simulink model "Calibration_IcestorageModel"  (R2018b)
settings: Solver=ode45  StartTime=(-31+16)*24*3600*0  StopTime=(31+29+31+30+31+30+31+31)*24*3600 %23*24*3600  EnableMultiTasking=on
libraries: carnot x43
(part 1 of 2)
settings Model: SimulationMode=accelerator  Creator=drhf  LastModifiedBy=drhf
settings DataIOCC: SaveFormat=Array  SignalLoggingSaveFormat=ModelDataLogs  SaveOutput=off  SignalLogging=off  DSMLogging=off  SaveTime=off
settings OptimizationCC: ExpressionDepthLimit=2147483647  LifeSpan=inf
settings DebuggingCC: UnderspecifiedInitializationDetection=Classic  MergeDetectMultiDrivingBlocksExec=none  SolverPrmCheckMsg=warning  FcnCallInpInsideContextMsg=warning  StateNameClashWarn=warning  SFUnexpectedBacktrackingDiag=warning  SFNoUnconditionalDefaultTransitionDiag=warning  SFExecutionAtInitializationDiag=none
settings HardwareCC: ProdBitPerPointer=32  ProdBitPerSizeT=32  ProdBitPerPtrDiffT=32  ProdLargestAtomicFloat=None  ProdIntDivRoundTo=Undefined  ProdEndianess=Unspecified  ProdWordSize=32  ProdHWDeviceType=32-bit Generic
settings ModelReferenceCC: PropagateSignalLabelsOutOfModel=off
settings SFSimCC: SimUseLocalCustomCode=off
settings RTWCC: RTWUseLocalCustomCode=off
settings CodeAppCC: StateflowObjectComments=on
settings GRTTargetCC: TargetLangStandard=C89/C90 (ANSI)  GeneratePreprocessorConditionals=Disable all  CombineOutputUpdateFcns=off  GRTInterface=on
settings ConfigComp: CovMetricSettings=dw  CovHtmlReporting=on  CovSaveCumulativeToWorkspaceVar=on  CovSaveSingleToWorkspaceVar=on  CovExternalEMLEnable=off

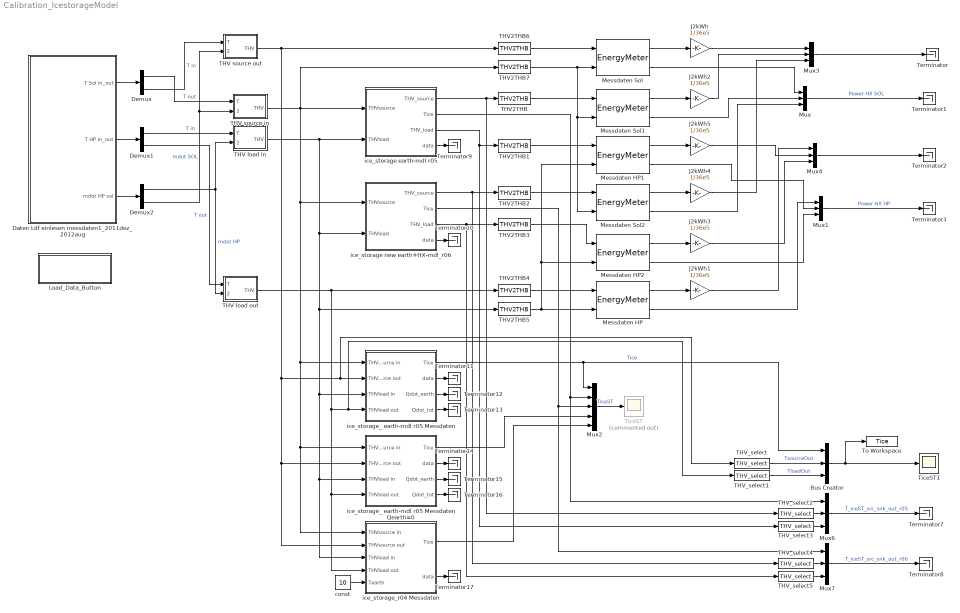
== system Calibration_IcestorageModel ==
  Bus Creator : BusCreator  Inputs=3
  Daten Ldf einlesen messdaten1_2011dez_2012aug : Subsystem
  Demux : Demux  Outputs=2
  Demux1 : Demux  Outputs=2
  Demux2 : Demux  Outputs=2
  J2kWh{,1..5} (6 alike) : Gain  Gain=1/36e5  SaturateOnIntegerOverflow=on  OutDataTypeStr=Inherit: Same as input  ParamDataTypeStr=Inherit: Same as input
  Load_Data_Button : Subsystem
      settings: OpenFcn=|
      | [filename, pathname, filterindex] = ...
      |    uigetfile( {'*.mat','MAT-files (*.mat)'; ...
      |    '*.*',  'All Files (*.*)'},  'Pick a data file');
      | 
      | if (filterindex > 0)
      |    load(filename)
      | end
      mask Display: disp('double click \nto load data')
  Messdaten HP : carnot/Control/EnergyMeter
      settings: SourceProductName=Carnot
  Messdaten HP1 : carnot/Control/EnergyMeter
      settings: SourceProductName=Carnot
  Messdaten HP2 : carnot/Control/EnergyMeter
      settings: SourceProductName=Carnot
  Messdaten Sol : carnot/Control/EnergyMeter
      settings: SourceProductName=Carnot
  Messdaten Sol1 : carnot/Control/EnergyMeter
      settings: SourceProductName=Carnot
  Messdaten Sol2 : carnot/Control/EnergyMeter
      settings: SourceProductName=Carnot
  Mux{,1,3..4,6..7} (6 alike) : Mux  Inputs=3
  Mux2 : Mux  Inputs=5
  THV load in : Subsystem  mask(create THV){p=1e5, fluid=water_glycol_mix, mix=0.5, dia=0.025}
      mask prompts: p "pressure [Pa]"; mix "fluid mixture [0..1]"; dia "diameter [m]"
      mask help: Block to create a THV vector with the variable input T and mdot. The other value can be set as constants in the mask.
      mask init:
      | mix = min(1, max(0, mix));
      | dia = max(dia, 0.001);
      mask Help: eval('man (''create_THV'')')
      mask TypeOptions fluid: water | air | cotton_oil | silicone_oil | water_glycol_mix
  THV load out : Subsystem  mask(create THV){p=1e5, fluid=water_glycol_mix, mix=0.5, dia=0.025}
      mask prompts: p "pressure [Pa]"; mix "fluid mixture [0..1]"; dia "diameter [m]"
      mask help: Block to create a THV vector with the variable input T and mdot. The other value can be set as constants in the mask.
      mask init:
      | mix = min(1, max(0, mix));
      | dia = max(dia, 0.001);
      mask Help: eval('man (''create_THV'')')
      mask TypeOptions fluid: water | air | cotton_oil | silicone_oil | water_glycol_mix
  THV source in : Subsystem  mask(create THV){p=1e5, fluid=water_glycol_mix, mix=0.5, dia=0.025}
      mask prompts: p "pressure [Pa]"; mix "fluid mixture [0..1]"; dia "diameter [m]"
      mask help: Block to create a THV vector with the variable input T and mdot. The other value can be set as constants in the mask.
      mask init:
      | mix = min(1, max(0, mix));
      | dia = max(dia, 0.001);
      mask Help: eval('man (''create_THV'')')
      mask TypeOptions fluid: water | air | cotton_oil | silicone_oil | water_glycol_mix
  THV source out : Subsystem  mask(create THV){p=1e5, fluid=water_glycol_mix, mix=0.5, dia=0.025}
      mask prompts: p "pressure [Pa]"; mix "fluid mixture [0..1]"; dia "diameter [m]"
      mask help: Block to create a THV vector with the variable input T and mdot. The other value can be set as constants in the mask.
      mask init:
      | mix = min(1, max(0, mix));
      | dia = max(dia, 0.001);
      mask Help: eval('man (''create_THV'')')
      mask TypeOptions fluid: water | air | cotton_oil | silicone_oil | water_glycol_mix
  THV2THB{,1..7} (8 alike) : carnot/Toolbox/THV2THB
      settings: SourceProductName=Carnot
  THV_select{,1..5} (6 alike) : carnot/Outputs/THV_select  f=off  t=on  m=off  p=off  id=off  mix=off  d=off  dpcon=off  dplin=off  dpqua=off
      settings: SourceProductName=Carnot
  Terminator{,1..3,7..17} (15 alike) : Terminator
  TiceST : Scope  Commented=on
  TiceST1 : Scope
  To Workspace : ToWorkspace  VariableName=Tice  SaveFormat=Timeseries  SampleTime=600
  const : Constant  Value=10
  ice_storage earth-mdl r05 : Subsystem  mask(simple water storage){vol=10, l_solar=30*3, l_hp=8*40, f_ice=0.075, t_ini=0, z=3.32-0.12, h=2.3, dearth=1, Tmeanoutside=11, deltathetae=9.3, Tmeaninside=5, deltathetai=15, tshift=319 %+8760/2 %to get the right behaviour!, cond_ground=2, cp_ground=800, rho_ground=2500}
      mask prompts: vol "volume [m³]"; l_solar "length of solar heat exchanger [m]"; l_hp "length of HP heat exchanger [m]"; f_ice "Initial fraction of ice (0..1)"; t_ini "Initial Temperatur (only if fraction ice = 0) [°C]"; z "depth of baseplate from upper surface [m]"; h "height of ice storage [m]"; dearth "thickness of surrounding earth layer [m]"; Tmeanoutside "mean outside temperature over one year [°C]"; deltathetae "amplitude of monthly outside temperatures [°C]"; Tmeaninside "mean inside temperature over one year [°C]"; deltathetai "amplitude of monthly mean inside temperature [°C]"; tshift "time shift where external temperature sine-curve shows a minimum [h]"; cond_ground "conductivity of ground [W/(m*K)]"; cp_ground "capacity of ground [J/(kg*K)]"; rho_ground "density of ground [kg/m^3]"
      mask help: multinode water storage
      mask init:
      | f_ice = min(1, max(0, f_ice));
      | h_ini = (1-f_ice)*335e3;
      | if f_ice == 0 
      |     h_ini = h_ini + 4182*t_ini;
      | end
      | %Durchmesser Eisspeicher [m]
      | D_tank = 2.7;
      | %Höhe Eisspeicher [m]
      | h_tank = 2.3;
      | %Grundfläche [m^2]
      | A = pi*(D_tank/2.)^2;
      | %Umfang [m]
      | P = D_tank*pi;
      | %charakteristisches Bodenmass [m]
      | B = A/(0.5*P);
      | %Wärmewiderstand Boden & Wand [m^2*K/W]
      | Rbtot = 0.12/1.330;
      | Rwtot = 0.1/1.330;
      | %Wanddicke [m]
      | w = 0.1;
      | %wirksame Dicke Boden & Wand [m]
      | dt = w + cond_ground*Rbtot;
      | dw = cond_ground*Rwtot;
      | %abstand der mitte der wandfläche zur oberfläche [m]
      | ztilde = z-(0.5*h);
      | %anzahl stunden pro jahr
      | t0 = 8760;
      | %thermische eindringtiefe
      | delta_grd = sqrt((t0*3600*cond_ground)/(pi*rho_ground*cp_ground));
      | 
      | %U-Wert Erdschicht [W/m^2K]
      | U_earth = cond_ground/dearth;
      | %Oberfläche Erdschicht [m^2]
      | A_earth = ((D_tank+2*dearth)/2)^2*pi + (D_tank+2*dearth)*pi*(h_tank+dearth);
      | %Volumen Erdschicht [m^3]
      | V_earth = ((D_tank+2*dearth)/2)^2*pi*(h_tank+dearth) - (D_tank/2)^2*pi*h_tank;
      | %U*A tank
      | UA_tank = (D_tank/2)^2*pi/(0.12/1.330) + D_tank*pi*h_tank/(0.1/1.330);
      mask Help: eval('man(''storage'')')
      mask Display: plot(0,0,100,100,[20,30,40,50,60,70,70,60,50,40,30,20,20],[70,90,84,84,90,70,20,13,10,10,13,20,70],[60,50,40,30],[90,95,95,90],[70,60,50,40,30,20],[70,64,60,60,64,70],[45,45],[20,50],[56,35],[35,35],[53,37],[26,44],[53,37],[44,26],[48,45,42],[46,43,46],[54,51,54],[33,35,38],[48,45,42],[24,28,23],[37,40,37],[32,35,38])
  ice_storage new earth+HX-mdl_r06 : Subsystem  mask(simple water storage){vol=10, l_solar=30*3, l_hp=8*40, f_ice=0.075, t_ini=0, z=3.32-0.12, h=2.3, dearth=1, Tmeanoutside=11, deltathetae=9.3, Tmeaninside=5, deltathetai=15, tshift=319 %+8760/2 %to get the right behaviour!, cond_ground=2, cp_ground=800, rho_ground=2500}
      mask prompts: vol "volume [m³]"; l_solar "length of solar heat exchanger [m]"; l_hp "length of HP heat exchanger [m]"; f_ice "Initial fraction of ice (0..1)"; t_ini "Initial Temperatur (only if fraction ice = 0) [°C]"; z "depth of baseplate from upper surface [m]"; h "height of ice storage [m]"; dearth "thickness of surrounding earth layer [m]"; Tmeanoutside "mean outside temperature over one year [°C]"; deltathetae "amplitude of monthly outside temperatures [°C]"; Tmeaninside "mean inside temperature over one year [°C]"; deltathetai "amplitude of monthly mean inside temperature [°C]"; tshift "time shift where external temperature sine-curve shows a minimum [h]"; cond_ground "conductivity of ground [W/(m*K)]"; cp_ground "capacity of ground [J/(kg*K)]"; rho_ground "density of ground [kg/m^3]"
      mask help: multinode water storage
      mask init: same as Calibration_IcestorageModel/ice_storage earth-mdl r05
      mask Help: eval('man(''storage'')')
      mask Display: plot(0,0,100,100,[20,30,40,50,60,70,70,60,50,40,30,20,20],[70,90,84,84,90,70,20,13,10,10,13,20,70],[60,50,40,30],[90,95,95,90],[70,60,50,40,30,20],[70,64,60,60,64,70],[45,45],[20,50],[56,35],[35,35],[53,37],[26,44],[53,37],[44,26],[48,45,42],[46,43,46],[54,51,54],[33,35,38],[48,45,42],[24,28,23],[37,40,37],[32,35,38])
  ice_storage_ earth-mdl r05 Messdaten : Subsystem  mask(simple water storage){vol=10, l_solar=30*3, l_hp=8*40, f_ice=0.075, t_ini=0, z=3.32-0.12, h=2.3, dearth=1, Tmeanoutside=11, deltathetae=9.3, Tmeaninside=5, deltathetai=15, tshift=319 %+8760/2 %to get the right behaviour!, cond_ground=2, cp_ground=800, rho_ground=2500}
      mask prompts: vol "volume [m³]"; l_solar "length of solar heat exchanger [m]"; l_hp "length of HP heat exchanger [m]"; f_ice "Initial fraction of ice (0..1)"; t_ini "Initial Temperatur (only if fraction ice = 0) [°C]"; z "depth of baseplate from upper surface [m]"; h "height of ice storage [m]"; dearth "thickness of surrounding earth layer [m]"; Tmeanoutside "mean outside temperature over one year [°C]"; deltathetae "amplitude of monthly outside temperatures [°C]"; Tmeaninside "mean inside temperature over one year [°C]"; deltathetai "amplitude of monthly mean inside temperature [°C]"; tshift "time shift where external temperature sine-curve shows a minimum [h]"; cond_ground "conductivity of ground [W/(m*K)]"; cp_ground "capacity of ground [J/(kg*K)]"; rho_ground "density of ground [kg/m^3]"
      mask help: multinode water storage
      mask init: same as Calibration_IcestorageModel/ice_storage earth-mdl r05
      mask Help: eval('man(''storage'')')
      mask Display: plot(0,0,100,100,[20,30,40,50,60,70,70,60,50,40,30,20,20],[70,90,84,84,90,70,20,13,10,10,13,20,70],[60,50,40,30],[90,95,95,90],[70,60,50,40,30,20],[70,64,60,60,64,70],[45,45],[20,50],[56,35],[35,35],[53,37],[26,44],[53,37],[44,26],[48,45,42],[46,43,46],[54,51,54],[33,35,38],[48,45,42],[24,28,23],[37,40,37],[32,35,38])
  ice_storage_ earth-mdl r05 Messdaten Qearth=0 : Subsystem  mask(simple water storage){vol=10, l_solar=30*3, l_hp=8*40, f_ice=0.075, t_ini=0, z=3.32-0.12, h=2.3, dearth=1, Tmeanoutside=11, deltathetae=9.3, Tmeaninside=5, deltathetai=15, tshift=319 %+8760/2 %to get the right behaviour!, cond_ground=2, cp_ground=800, rho_ground=2500}
      mask prompts: vol "volume [m³]"; l_solar "length of solar heat exchanger [m]"; l_hp "length of HP heat exchanger [m]"; f_ice "Initial fraction of ice (0..1)"; t_ini "Initial Temperatur (only if fraction ice = 0) [°C]"; z "depth of baseplate from upper surface [m]"; h "height of ice storage [m]"; dearth "thickness of surrounding earth layer [m]"; Tmeanoutside "mean outside temperature over one year [°C]"; deltathetae "amplitude of monthly outside temperatures [°C]"; Tmeaninside "mean inside temperature over one year [°C]"; deltathetai "amplitude of monthly mean inside temperature [°C]"; tshift "time shift where external temperature sine-curve shows a minimum [h]"; cond_ground "conductivity of ground [W/(m*K)]"; cp_ground "capacity of ground [J/(kg*K)]"; rho_ground "density of ground [kg/m^3]"
      mask help: multinode water storage
      mask init: same as Calibration_IcestorageModel/ice_storage earth-mdl r05
      mask Help: eval('man(''storage'')')
      mask Display: plot(0,0,100,100,[20,30,40,50,60,70,70,60,50,40,30,20,20],[70,90,84,84,90,70,20,13,10,10,13,20,70],[60,50,40,30],[90,95,95,90],[70,60,50,40,30,20],[70,64,60,60,64,70],[45,45],[20,50],[56,35],[35,35],[53,37],[26,44],[53,37],[44,26],[48,45,42],[46,43,46],[54,51,54],[33,35,38],[48,45,42],[24,28,23],[37,40,37],[32,35,38])
  ice_storage_r04 Messdaten : Subsystem  mask(simple water storage){vol=10, l_solar=30*3, l_hp=8*40, f_ice=0.075, t_ini=0}
      mask prompts: vol "volume in m³"; l_solar "length of solar heat exchanger in m"; l_hp "length of HP heat exchanger in m"; f_ice "Initial fraction of ice (0..1)"; t_ini "Initial Temperatur (only if fraction ice = 0) in °C"
      mask help: multinode water storage
      mask init:
      | f_ice = min(1, max(0, f_ice));
      | h_ini = (1-f_ice)*335e3;
      | if f_ice == 0 
      |     h_ini = h_ini + 4182*t_ini;
      | end
      mask Help: eval('man(''storage'')')
      mask Display: plot(0,0,100,100,[20,30,40,50,60,70,70,60,50,40,30,20,20],[70,90,84,84,90,70,20,13,10,10,13,20,70],[60,50,40,30],[90,95,95,90],[70,60,50,40,30,20],[70,64,60,60,64,70],[45,45],[20,50],[56,35],[35,35],[53,37],[26,44],[53,37],[44,26],[48,45,42],[46,43,46],[54,51,54],[33,35,38],[48,45,42],[24,28,23],[37,40,37],[32,35,38])
  wires:
  THV load in/1(THV) -> ice_storage earth-mdl r05/2(THVload), THV2THB5/1, ice_storage_ earth-mdl r05 Messdaten/3(THVload in), ice_storage_ earth-mdl r05 Messdaten Qearth=0/3(THVload in), ice_storage_r04 Messdaten/3(THVload in), ice_storage new earth+HX-mdl_r06/2(THVload)
  Daten Ldf einlesen messdaten1_2011dez_2012aug/1(T Sol in_out) -> Demux/1
  Daten Ldf einlesen messdaten1_2011dez_2012aug/2(T HP in_out) -> Demux1/1
  Daten Ldf einlesen messdaten1_2011dez_2012aug/3(mdot HP sol) -> Demux2/1
  Demux/1 -> THV source in/1(T)  "T out"
  Demux/2 -> THV source out/1(T)  "T in"
  Demux1/2 -> THV load out/1(T)  "T out"
  Demux2/1 -> THV load in/2(mvdot), THV load out/2(mvdot)  "mdot HP"
  Demux2/2 -> THV source out/2(mvdot), THV source in/2(mvdot)  "mdot SOL"
  THV source in/1(THV) -> ice_storage earth-mdl r05/1(THVsource), THV2THB7/1, ice_storage new earth+HX-mdl_r06/1(THVsource), ice_storage_ earth-mdl r05 Messdaten/1(THVsource in), ice_storage_ earth-mdl r05 Messdaten Qearth=0/1(THVsource in), ice_storage_r04 Messdaten/1(THVsource in)
  THV load out/1(THV) -> THV2THB4/1, ice_storage_ earth-mdl r05 Messdaten Qearth=0/4(THVload out), ice_storage_r04 Messdaten/4(THVload out), ice_storage_ earth-mdl r05 Messdaten/4(THVload out), THV_select1/1
  Messdaten Sol/1 -> J2kWh/1
  Messdaten HP/1 -> J2kWh1/1
  ice_storage earth-mdl r05/1(THV_source) -> THV2THB/1, THV_select2/1
  Messdaten Sol1/1 -> J2kWh2/1
  ice_storage earth-mdl r05/3(THV_load) -> THV2THB1/1, THV_select3/1
  ice_storage new earth+HX-mdl_r06/1(THV_source) -> THV_select4/1, THV2THB2/1
  ice_storage new earth+HX-mdl_r06/3(THV_load) -> THV_select5/1, THV2THB3/1
  Messdaten HP1/1 -> J2kWh5/1
  Messdaten Sol2/1 -> J2kWh4/1
  Messdaten HP2/1 -> J2kWh3/1
  Messdaten Sol/2 -> Mux/1
  Messdaten Sol1/2 -> Mux/2
  Messdaten Sol2/2 -> Mux/3
  Messdaten HP2/2 -> Mux1/3
  Messdaten HP1/2 -> Mux1/2
  Mux/1 -> Terminator1/1  "Power HX SOL"
  Mux1/1 -> Terminator3/1  "Power HX HP"
  Messdaten HP/2 -> Mux1/1
  ice_storage earth-mdl r05/2(Tice) -> Mux2/2, Mux6/1
  ice_storage new earth+HX-mdl_r06/2(Tice) -> Mux2/3, Mux7/1
  Mux2/1 -> TiceST/1  "TiceST"
  ice_storage_ earth-mdl r05 Messdaten/1(Tice) -> Bus Creator/1, Mux2/1  "Tice"
  ice_storage_ earth-mdl r05 Messdaten Qearth=0/1(Tice) -> Mux2/4
  ice_storage_r04 Messdaten/1(Tice) -> Mux2/5
  const/1 -> ice_storage_r04 Messdaten/5(Tearth)
  Mux3/1 -> Terminator/1
  J2kWh/1 -> Mux3/1
  J2kWh2/1 -> Mux3/2
  J2kWh4/1 -> Mux3/3
  Mux4/1 -> Terminator2/1
  J2kWh1/1 -> Mux4/1
  J2kWh5/1 -> Mux4/2
  J2kWh3/1 -> Mux4/3
  Bus Creator/1 -> TiceST1/1, To Workspace/1
  THV_select/1 -> Bus Creator/2  "TsourceOut"
  THV_select1/1 -> Bus Creator/3  "TloadOut"
  Mux6/1 -> Terminator7/1  "T_iceST_src_snk_out_r05"
  Mux7/1 -> Terminator8/1  "T_iceST_src_snk_out_r06"
  THV_select2/1 -> Mux6/2
  THV_select3/1 -> Mux6/3
  THV_select4/1 -> Mux7/2
  THV_select5/1 -> Mux7/3
  Demux1/1 -> THV load in/1(T)  "T in"
  ice_storage earth-mdl r05/4(data) -> Terminator9/1
  ice_storage new earth+HX-mdl_r06/4(data) -> Terminator10/1
  ice_storage_ earth-mdl r05 Messdaten/2(data) -> Terminator11/1
  ice_storage_ earth-mdl r05 Messdaten/3(Qdot_earth) -> Terminator12/1
  ice_storage_ earth-mdl r05 Messdaten/4(Qdot_tot) -> Terminator13/1
  ice_storage_ earth-mdl r05 Messdaten Qearth=0/2(data) -> Terminator14/1
  ice_storage_ earth-mdl r05 Messdaten Qearth=0/3(Qdot_earth) -> Terminator15/1
  ice_storage_ earth-mdl r05 Messdaten Qearth=0/4(Qdot_tot) -> Terminator16/1
  ice_storage_r04 Messdaten/2(data) -> Terminator17/1
  THV2THB/1 -> Messdaten Sol1/1
  THV2THB1/1 -> Messdaten HP1/1
  THV2THB2/1 -> Messdaten Sol2/1
  THV2THB3/1 -> Messdaten HP2/1
  THV2THB4/1 -> Messdaten HP/1
  THV2THB5/1 -> Messdaten HP/2, Messdaten HP1/2, Messdaten HP2/2
  THV source out/1(THV) -> THV2THB6/1, ice_storage_ earth-mdl r05 Messdaten Qearth=0/2(THVsource out), ice_storage_r04 Messdaten/2(THVsource out), ice_storage_ earth-mdl r05 Messdaten/2(THVsource out), THV_select/1
  THV2THB6/1 -> Messdaten Sol/1
  THV2THB7/1 -> Messdaten Sol/2, Messdaten Sol1/2, Messdaten Sol2/2

== system Calibration_IcestorageModel/Daten Ldf einlesen messdaten1_2011dez_2012aug ==
  From Workspace : FromWorkspace  VariableName=messdaten1_2011dez_2012aug  SampleTime=60  Interpolate=off  OutputAfterFinalValue=Holding final value
  Heiz : Subsystem  mask(Selector Messdaten Viessmann){a1=on, a2=off, a3=off, a4=off, a5=off, a6=off, a7=off, a8=off, a9=off, a10=off}
      mask prompts: a1 "Heizkreis_Wh [NONE]"; a2 "Heizkreis_m3 [NONE]"; a3 "Heizkreis_m3/h [NONE]"; a4 "Heizkreis_Tflow [NONE]"; a5 "Heizkreis_Treturn [NONE]"; a6 "TWW+Zirkulation_Wh [NONE]"; a7 "TWW+Zirkulation_m3 [NONE]"; a8 "TWW+Zirkulation_m3/h [NONE]"; a9 "TWW+Zirkulation_Tflow [NONE]"; a10 "TWW+Zirkulation_Treturn [NONE]"
      mask help:
      | Wählt die Messdaten der Viessmann Eisspeicher Anlage aus.
      | Daten der Messungen:
      | Dezember 2011 - August 2012
      mask init:
      | v=[];
      | if (a1)  v = [4];     end
      | if (a2)  v = [v 5];     end
      | if (a3)  v = [v 6];    end
      | if (a4)  v = [v 7];    end
      | if (a5)  v = [v 8];    end
      | if (a6)  v = [v 29];    end
      | if (a7)  v = [v 30];    end
      | if (a8)  v = [v 31];    end
      | if (a9)  v = [v 32];    end
      | if (a10)  v = [v 33];    end
      | if (~numel(v)) v = [6]; end
  InteressanterRest : Subsystem  mask(Selector Messdaten Viessmann){a1=on, a2=off, a3=off, a4=off, a5=off, a6=off, a7=off, a8=off, a9=off, a10=off, a11=off, a12=off, a13=off, a14=off}
      mask prompts: a1 "Einstrahlung [Ampere 4-20mA=0-1500W]"; a2 "Resol  Sol-Eis VL [Celsius]"; a3 "Resol Eis-WP [m^3]"; a4 "Resol Eis-WP RL [Celsius]"; a5 "Resol Eis-WP VL [Celsius]"; a6 "Resol Sol-Eis [m^3]"; a7 "Resol Sol-Eis RL [Celsius]"; a8 "Resol Sol-WP [m^3]"; a9 "Resol Sol-WP RL [Celsius]"; a10 "Resol Sol-WP VL [Celsius]"; a11 "RT Heizkeller [Celsius]"; a12 "Ventil R2_UmschKol [Volt]"; a13 "Ventil_R3_SolPumpe [Volt]"; a14 "Ventil_R4_UmschSpe [Volt]"
      mask help:
      | Wählt die Messdaten der Viessmann Eisspeicher Anlage aus.
      | Daten der Messungen:
      | Dezember 2011 - August 2012
      mask init:
      | v=[];
      | if (a1)  v = [3];     end
      | if (a2)  v = [v 9];     end
      | if (a3)  v = [v 10];    end
      | if (a4)  v = [v 11];    end
      | if (a5)  v = [v 12];    end
      | if (a6)  v = [v 13];    end
      | if (a7)  v = [v 14];     end
      | if (a8)  v = [v 15];     end
      | if (a9)  v = [v 16];    end
      | if (a10)  v = [v 17];    end
      | if (a11)  v = [v 18];    end
      | if (a12)  v = [v 34];    end
      | if (a13)  v = [v 35];     end
      | if (a14)  v = [v 36];     end
      | if (~numel(v)) v = [6]; end
  InteressanterRest1 : Subsystem  mask(Selector Messdaten Viessmann){a1=off, a2=on, a3=off, a4=off, a5=off, a6=off, a7=on, a8=off, a9=off, a10=off, a11=off, a12=off, a13=off, a14=off}
      mask prompts: a1 "Einstrahlung [Ampere 4-20mA=0-1500W]"; a2 "Resol  Sol-Eis VL [Celsius]"; a3 "Resol Eis-WP [m^3]"; a4 "Resol Eis-WP RL [Celsius]"; a5 "Resol Eis-WP VL [Celsius]"; a6 "Resol Sol-Eis [m^3]"; a7 "Resol Sol-Eis RL [Celsius]"; a8 "Resol Sol-WP [m^3]"; a9 "Resol Sol-WP RL [Celsius]"; a10 "Resol Sol-WP VL [Celsius]"; a11 "RT Heizkeller [Celsius]"; a12 "Ventil R2_UmschKol [Volt]"; a13 "Ventil_R3_SolPumpe [Volt]"; a14 "Ventil_R4_UmschSpe [Volt]"
      mask help:
      | Wählt die Messdaten der Viessmann Eisspeicher Anlage aus.
      | Daten der Messungen:
      | Dezember 2011 - August 2012
      mask init: same as Calibration_IcestorageModel/Daten Ldf einlesen messdaten1_2011dez_2012aug/InteressanterRest
  InteressanterRest2 : Subsystem  mask(Selector Messdaten Viessmann){a1=off, a2=off, a3=off, a4=on, a5=on, a6=off, a7=off, a8=off, a9=off, a10=off, a11=off, a12=off, a13=off, a14=off}
      mask prompts: a1 "Einstrahlung [Ampere 4-20mA=0-1500W]"; a2 "Resol  Sol-Eis VL [Celsius]"; a3 "Resol Eis-WP [m^3]"; a4 "Resol Eis-WP RL [Celsius]"; a5 "Resol Eis-WP VL [Celsius]"; a6 "Resol Sol-Eis [m^3]"; a7 "Resol Sol-Eis RL [Celsius]"; a8 "Resol Sol-WP [m^3]"; a9 "Resol Sol-WP RL [Celsius]"; a10 "Resol Sol-WP VL [Celsius]"; a11 "RT Heizkeller [Celsius]"; a12 "Ventil R2_UmschKol [Volt]"; a13 "Ventil_R3_SolPumpe [Volt]"; a14 "Ventil_R4_UmschSpe [Volt]"
      mask help:
      | Wählt die Messdaten der Viessmann Eisspeicher Anlage aus.
      | Daten der Messungen:
      | Dezember 2011 - August 2012
      mask init: same as Calibration_IcestorageModel/Daten Ldf einlesen messdaten1_2011dez_2012aug/InteressanterRest
  InteressanterRest3 : Subsystem  mask(Selector Messdaten Viessmann){a1=off, a2=off, a3=on, a4=off, a5=off, a6=on, a7=off, a8=off, a9=off, a10=off, a11=off, a12=off, a13=off, a14=off}
      mask prompts: a1 "Einstrahlung [Ampere 4-20mA=0-1500W]"; a2 "Resol  Sol-Eis VL [Celsius]"; a3 "Resol Eis-WP [m^3]"; a4 "Resol Eis-WP RL [Celsius]"; a5 "Resol Eis-WP VL [Celsius]"; a6 "Resol Sol-Eis [m^3]"; a7 "Resol Sol-Eis RL [Celsius]"; a8 "Resol Sol-WP [m^3]"; a9 "Resol Sol-WP RL [Celsius]"; a10 "Resol Sol-WP VL [Celsius]"; a11 "RT Heizkeller [Celsius]"; a12 "Ventil R2_UmschKol [Volt]"; a13 "Ventil_R3_SolPumpe [Volt]"; a14 "Ventil_R4_UmschSpe [Volt]"
      mask help:
      | Wählt die Messdaten der Viessmann Eisspeicher Anlage aus.
      | Daten der Messungen:
      | Dezember 2011 - August 2012
      mask init: same as Calibration_IcestorageModel/Daten Ldf einlesen messdaten1_2011dez_2012aug/InteressanterRest
  Strom : Subsystem  mask(Selector Messdaten Viessmann){a1=off, a2=on, a3=off, a4=off, a5=off, a6=off}
      mask prompts: a1 "Drehstrom E-Heizst [kWh]"; a2 "Drestrom WP [kWh]"; a3 "Strom Primärpumpe [kWh]"; a4 "Strom Regelung [kWh]"; a5 "Strom Sekundärpump [kWh]"; a6 "Strom Solarstation [NONE]"
      mask help:
      | Wählt die Messdaten der Viessmann Eisspeicher Anlage aus.
      | Daten der Messungen:
      | Dezember 2011 - August 2012
      mask init:
      | v=[];
      | if (a1)  v = [1];     end
      | if (a2)  v = [v 2];     end
      | if (a3)  v = [v 19];    end
      | if (a4)  v = [v 20];    end
      | if (a5)  v = [v 21];    end
      | if (a6)  v = [v 22];    end
      | if (~numel(v)) v = [6]; end
  THO : Subsystem  mask(Selector Messdaten Viessmann){a1=on, a2=off, a3=off, a4=off, a5=off, a6=off}
      mask prompts: a1 "THO_rhoinst [NONE]"; a2 "THO_rhomax [NONE]"; a3 "THO_rhomin [NONE]"; a4 "THO_Tinst [NONE]"; a5 "THO_Tmax [NONE]"; a6 "THO_Tmin [NONE]"
      mask help:
      | Wählt die Messdaten der Viessmann Eisspeicher Anlage aus.
      | Daten der Messungen:
      | Dezember 2011 - August 2012
      mask init:
      | v=[];
      | if (a1)  v = [23];     end
      | if (a2)  v = [v 24];     end
      | if (a3)  v = [v 25];    end
      | if (a4)  v = [v 26];    end
      | if (a5)  v = [v 27];    end
      | if (a6)  v = [v 28];    end
      | if (~numel(v)) v = [6]; end
  Terminator{,1..3} (4 alike) : Terminator
  converts 4-20mA  to  0-1500W : Subsystem
  T Sol in_out : Outport
  T HP in_out : Outport  Port=2
  mdot HP sol : Outport  Port=3
  wires:
  THO/1(out) -> Terminator1/1
  Heiz/1(out) -> Terminator/1
  converts 4-20mA  to  0-1500W/1(Out1) -> Terminator3/1
  InteressanterRest/1(out) -> converts 4-20mA  to  0-1500W/1(In1)
  Strom/1(out) -> Terminator2/1
  From Workspace/1 -> InteressanterRest1/1(data), InteressanterRest2/1(data), InteressanterRest3/1(data), InteressanterRest/1(data), THO/1(data), Heiz/1(data), Strom/1(data)
  InteressanterRest1/1(out) -> T Sol in_out/1
  InteressanterRest2/1(out) -> T HP in_out/1
  InteressanterRest3/1(out) -> mdot HP sol/1

== system Calibration_IcestorageModel/Load_Data_Button ==

== system Calibration_IcestorageModel/THV load in ==
  note: mdot
  T : Inport
  mvdot : Inport  Port=2
  Gain : Gain  Gain=1/60
  Ground : Ground
  Mux1 : Mux  Inputs=[1 1 1 4 13]
  Product : Product  RndMeth=Zero
  const : Constant
  const1 : Constant  Value=[p fluid mix dia]
  const2 : Constant  Value=p
  const3 : Constant  Value=fluid
  const4 : Constant  Value=mix
  density : carnot/Basic/Material_Properties/Density  VariantControl=CarlibClassic  INPUTARGUMENTS=state variables (classic)  DEBUGLEVEL=DEBUGLEVEL  MAXTOTALWARNINGS=inf  MAXCONSECUTIVEWARNINGS=inf  WRITETOFILE=0  FILENAME='errors.txt'
      settings: SourceProductName=Carnot
  THV : Outport  InitialOutput=0
  wires:
  const1/1 -> Mux1/4
  T/1 -> Mux1/2, density/1
  Ground/1 -> Mux1/5
  const/1 -> Mux1/1
  Mux1/1 -> THV/1
  const2/1 -> density/2
  const3/1 -> density/3
  const4/1 -> density/4
  density/1 -> Product/1
  mvdot/1 -> Product/2
  Product/1 -> Gain/1
  Gain/1 -> Mux1/3

== system Calibration_IcestorageModel/THV load out ==
  note: mdot
  T : Inport
  mvdot : Inport  Port=2
  Gain : Gain  Gain=1/60
  Ground : Ground
  Mux1 : Mux  Inputs=[1 1 1 4 13]
  Product : Product  RndMeth=Zero
  const : Constant
  const1 : Constant  Value=[p fluid mix dia]
  const2 : Constant  Value=p
  const3 : Constant  Value=fluid
  const4 : Constant  Value=mix
  density : carnot/Basic/Material_Properties/Density  VariantControl=CarlibClassic  INPUTARGUMENTS=state variables (classic)  DEBUGLEVEL=DEBUGLEVEL  MAXTOTALWARNINGS=inf  MAXCONSECUTIVEWARNINGS=inf  WRITETOFILE=0  FILENAME='errors.txt'
      settings: SourceProductName=Carnot
  THV : Outport  InitialOutput=0
  wires:
  Gain/1 -> Mux1/3
  Product/1 -> Gain/1
  mvdot/1 -> Product/2
  density/1 -> Product/1
  const4/1 -> density/4
  const3/1 -> density/3
  const2/1 -> density/2
  Mux1/1 -> THV/1
  const/1 -> Mux1/1
  Ground/1 -> Mux1/5
  T/1 -> density/1, Mux1/2
  const1/1 -> Mux1/4

== system Calibration_IcestorageModel/THV source in ==
  note: mdot
  T : Inport
  mvdot : Inport  Port=2
  Gain : Gain  Gain=1/60
  Ground : Ground
  Mux1 : Mux  Inputs=[1 1 1 4 13]
  Product : Product  RndMeth=Zero
  const : Constant
  const1 : Constant  Value=[p fluid mix dia]
  const2 : Constant  Value=p
  const3 : Constant  Value=fluid
  const4 : Constant  Value=mix
  density : carnot/Basic/Material_Properties/Density  VariantControl=CarlibClassic  INPUTARGUMENTS=state variables (classic)  DEBUGLEVEL=DEBUGLEVEL  MAXTOTALWARNINGS=inf  MAXCONSECUTIVEWARNINGS=inf  WRITETOFILE=0  FILENAME='errors.txt'
      settings: SourceProductName=Carnot
  THV : Outport  InitialOutput=0
  wires:
  Gain/1 -> Mux1/3
  Product/1 -> Gain/1
  mvdot/1 -> Product/2
  density/1 -> Product/1
  const4/1 -> density/4
  const3/1 -> density/3
  const2/1 -> density/2
  Mux1/1 -> THV/1
  const/1 -> Mux1/1
  Ground/1 -> Mux1/5
  T/1 -> density/1, Mux1/2
  const1/1 -> Mux1/4

== system Calibration_IcestorageModel/THV source out ==
  note: mdot
  T : Inport
  mvdot : Inport  Port=2
  Gain : Gain  Gain=1/60
  Ground : Ground
  Mux1 : Mux  Inputs=[1 1 1 4 13]
  Product : Product  RndMeth=Zero
  const : Constant
  const1 : Constant  Value=[p fluid mix dia]
  const2 : Constant  Value=p
  const3 : Constant  Value=fluid
  const4 : Constant  Value=mix
  density : carnot/Basic/Material_Properties/Density  VariantControl=CarlibClassic  INPUTARGUMENTS=state variables (classic)  DEBUGLEVEL=DEBUGLEVEL  MAXTOTALWARNINGS=inf  MAXCONSECUTIVEWARNINGS=inf  WRITETOFILE=0  FILENAME='errors.txt'
      settings: SourceProductName=Carnot
  THV : Outport  InitialOutput=0
  wires:
  const1/1 -> Mux1/4
  T/1 -> Mux1/2, density/1
  Ground/1 -> Mux1/5
  const/1 -> Mux1/1
  Mux1/1 -> THV/1
  const2/1 -> density/2
  const3/1 -> density/3
  const4/1 -> density/4
  density/1 -> Product/1
  mvdot/1 -> Product/2
  Product/1 -> Gain/1
  Gain/1 -> Mux1/3

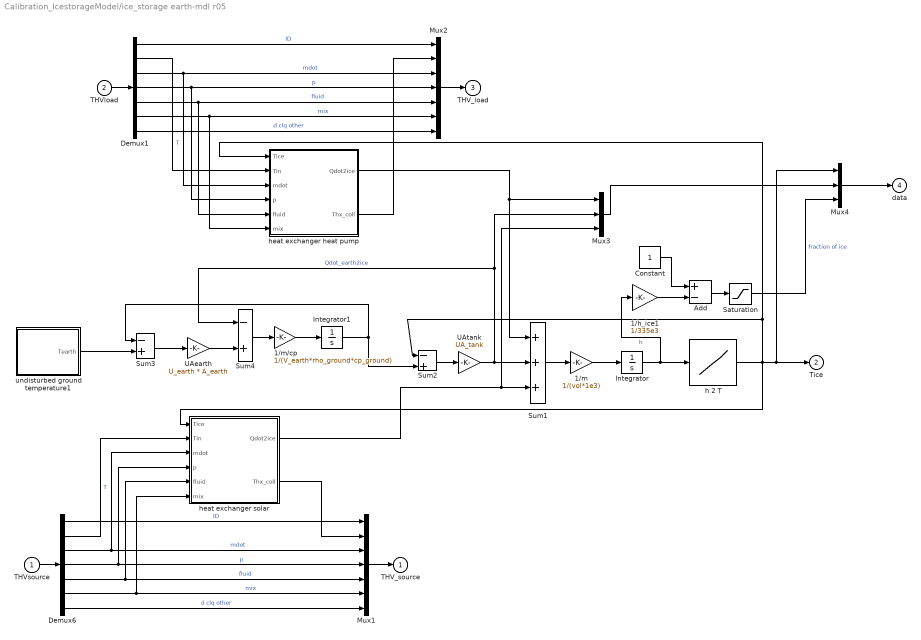
== system Calibration_IcestorageModel/ice_storage earth-mdl r05 ==
  THVsource : Inport
  THVload : Inport  Port=2
  1/h_ice1 : Gain  Gain=1/335e3  SaturateOnIntegerOverflow=on  OutDataTypeStr=Inherit: Same as input  ParamDataTypeStr=Inherit: Same as input
  1/m : Gain  Gain=1/(vol*1e3)  SaturateOnIntegerOverflow=on  OutDataTypeStr=Inherit: Same as input  ParamDataTypeStr=Inherit: Same as input
  1/m/cp : Gain  Gain=1/(V_earth*rho_ground*cp_ground)  SaturateOnIntegerOverflow=on  OutDataTypeStr=Inherit: Same as input  ParamDataTypeStr=Inherit: Same as input
  Add : Sum  Inputs=+-
  Constant : Constant
  Demux1 : Demux  Outputs=[1 1 1 1 1 1 14]
  Demux6 : Demux  Outputs=[1 1 1 1 1 1 14]
  Integrator : Integrator  InitialCondition=h_ini
  Integrator1 : Integrator  InitialCondition=5
  Mux1 : Mux  Inputs=7
  Mux2 : Mux  Inputs=7
  Mux3 : Mux  Inputs=3
  Mux4 : Mux  Inputs=3
  Saturation : Saturate  UpperLimit=1  LowerLimit=0  LinearizeAsGain=off
  Sum1 : Sum  Inputs=+++  SaturateOnIntegerOverflow=on  InputSameDT=on  OutDataTypeStr=Inherit: Same as first input
  Sum2 : Sum  Inputs=-+  SaturateOnIntegerOverflow=on  InputSameDT=on  OutDataTypeStr=Inherit: Same as first input
  Sum3 : Sum  Inputs=-+  SaturateOnIntegerOverflow=on  InputSameDT=on  OutDataTypeStr=Inherit: Same as first input
  Sum4 : Sum  Inputs=-+  SaturateOnIntegerOverflow=on  InputSameDT=on  OutDataTypeStr=Inherit: Same as first input
  UAearth : Gain  Gain=U_earth * A_earth  SaturateOnIntegerOverflow=on  OutDataTypeStr=Inherit: Same as input  ParamDataTypeStr=Inherit: Same as input
  UAtank : Gain  Gain=UA_tank  SaturateOnIntegerOverflow=on  OutDataTypeStr=Inherit: Same as input  ParamDataTypeStr=Inherit: Same as input
  h 2 T : Lookup  InputValues=[-2060*10 -2060*3 335e3 335e3+4182*10]  Table=[-10 -3 0 10]
  heat exchanger heat pump : Subsystem
  heat exchanger solar : Subsystem
  undisturbed ground temperature1 : Subsystem
  THV_source : Outport  InitialOutput=0
  Tice : Outport  Port=2  InitialOutput=0
  THV_load : Outport  Port=3  InitialOutput=0
  data : Outport  Port=4  InitialOutput=0
  wires:
  Mux3/1 -> Mux4/2
  heat exchanger heat pump/1(Qdot2ice) -> Mux3/1, Sum1/1
  heat exchanger heat pump/2(Thx_coll) -> Mux2/2
  Demux1/2 -> heat exchanger heat pump/2(Tin)  "T"
  Demux1/6 -> Mux2/6, heat exchanger heat pump/6(mix)  "mix"
  Demux1/1 -> Mux2/1  "ID"
  Demux1/7 -> Mux2/7  "d clq other"
  Demux1/5 -> Mux2/5, heat exchanger heat pump/5(fluid)  "fluid"
  Demux1/4 -> Mux2/4, heat exchanger heat pump/4(p)  "p"
  Demux1/3 -> Mux2/3, heat exchanger heat pump/3(mdot)  "mdot"
  Mux2/1 -> THV_load/1
  THVload/1 -> Demux1/1
  heat exchanger solar/1(Qdot2ice) -> Sum1/3, Mux3/3
  h 2 T/1 -> Sum2/1, heat exchanger heat pump/1(Tice), heat exchanger solar/1(Tice), Mux4/1, Tice/1
  Integrator1/1 -> Sum3/1, Sum2/2
  1/m/cp/1 -> Integrator1/1
  Sum4/1 -> 1/m/cp/1
  UAearth/1 -> Sum4/2
  Sum3/1 -> UAearth/1
  Integrator/1 -> h 2 T/1, 1/h_ice1/1  "h"
  UAtank/1 -> Mux3/2, Sum4/1, Sum1/2  "Qdot_earth2ice"
  Sum2/1 -> UAtank/1
  Sum1/1 -> 1/m/1
  1/m/1 -> Integrator/1
  heat exchanger solar/2(Thx_coll) -> Mux1/2
  Demux6/2 -> heat exchanger solar/2(Tin)  "T"
  Demux6/6 -> heat exchanger solar/6(mix), Mux1/6  "mix"
  Demux6/1 -> Mux1/1  "ID"
  Demux6/7 -> Mux1/7  "d clq other"
  Demux6/5 -> heat exchanger solar/5(fluid), Mux1/5  "fluid"
  Demux6/4 -> heat exchanger solar/4(p), Mux1/4  "p"
  Demux6/3 -> heat exchanger solar/3(mdot), Mux1/3  "mdot"
  Mux1/1 -> THV_source/1
  THVsource/1 -> Demux6/1
  Mux4/1 -> data/1
  1/h_ice1/1 -> Add/2
  Add/1 -> Saturation/1
  Constant/1 -> Add/1
  Saturation/1 -> Mux4/3  "fraction of ice"
  undisturbed ground temperature1/1(Tearth) -> Sum3/2

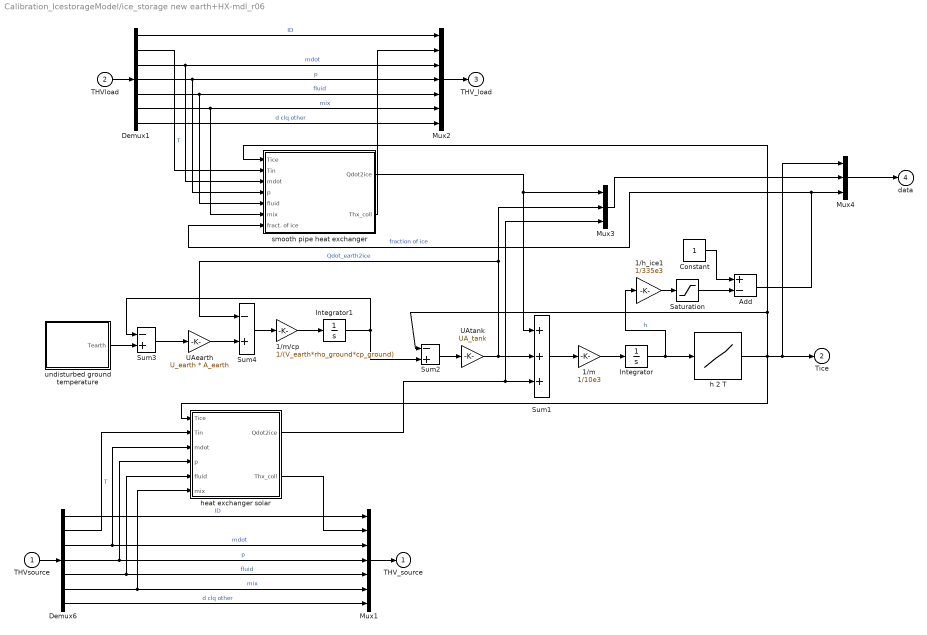
== system Calibration_IcestorageModel/ice_storage new earth+HX-mdl_r06 ==
  THVsource : Inport
  THVload : Inport  Port=2
  1/h_ice1 : Gain  Gain=1/335e3  SaturateOnIntegerOverflow=on  OutDataTypeStr=Inherit: Same as input  ParamDataTypeStr=Inherit: Same as input
  1/m : Gain  Gain=1/10e3  SaturateOnIntegerOverflow=on  OutDataTypeStr=Inherit: Same as input  ParamDataTypeStr=Inherit: Same as input
  1/m/cp : Gain  Gain=1/(V_earth*rho_ground*cp_ground)  SaturateOnIntegerOverflow=on  OutDataTypeStr=Inherit: Same as input  ParamDataTypeStr=Inherit: Same as input
  Add : Sum  Inputs=+-
  Constant : Constant
  Demux1 : Demux  Outputs=[1 1 1 1 1 1 14]
  Demux6 : Demux  Outputs=[1 1 1 1 1 1 14]
  Integrator : Integrator  InitialCondition=h_ini
  Integrator1 : Integrator  InitialCondition=5
  Mux1 : Mux  Inputs=7
  Mux2 : Mux  Inputs=7
  Mux3 : Mux  Inputs=3
  Mux4 : Mux  Inputs=3
  Saturation : Saturate  UpperLimit=1  LowerLimit=0  LinearizeAsGain=off
  Sum1 : Sum  Inputs=+++  SaturateOnIntegerOverflow=on  InputSameDT=on  OutDataTypeStr=Inherit: Same as first input
  Sum2 : Sum  Inputs=-+  SaturateOnIntegerOverflow=on  InputSameDT=on  OutDataTypeStr=Inherit: Same as first input
  Sum3 : Sum  Inputs=-+  SaturateOnIntegerOverflow=on  InputSameDT=on  OutDataTypeStr=Inherit: Same as first input
  Sum4 : Sum  Inputs=-+  SaturateOnIntegerOverflow=on  InputSameDT=on  OutDataTypeStr=Inherit: Same as first input
  UAearth : Gain  Gain=U_earth * A_earth  SaturateOnIntegerOverflow=on  OutDataTypeStr=Inherit: Same as input  ParamDataTypeStr=Inherit: Same as input
  UAtank : Gain  Gain=UA_tank  SaturateOnIntegerOverflow=on  OutDataTypeStr=Inherit: Same as input  ParamDataTypeStr=Inherit: Same as input
  h 2 T : Lookup  InputValues=[-2060*10 -2060*3 335e3 335e3+4182*10]  Table=[-10 -3 0 10]
  heat exchanger solar : Subsystem
  smooth pipe heat exchanger : Subsystem  mask{d_a=0.025, lhx=l_hp, dhxmat=0.0019, lambdahxmat=0.34}
      mask prompts: d_a "outer diameter of heat exchanger pipe [m]"; lhx "length of heat exchanger [m]"; dhxmat "thickness of heat exchanger material [m]"; lambdahxmat "thermal conductivity of pipe wall [W/mK]"
      mask init:
      | %inner diameter of pipe [m]
      | d_i = d_a - 2*dhxmat;
      | %heat exchanger surface [m^2]
      | Ahx = d_a*pi*lhx;
      | %heat transfer coefficient of pipe wall [W/m^2K]
      | uhxmat = lambdahxmat/dhxmat;
  undisturbed ground temperature : Subsystem
  THV_source : Outport  InitialOutput=0
  Tice : Outport  Port=2  InitialOutput=0
  THV_load : Outport  Port=3  InitialOutput=0
  data : Outport  Port=4  InitialOutput=0
  wires:
  smooth pipe heat exchanger/2(Thx_coll) -> Mux2/2
  smooth pipe heat exchanger/1(Qdot2ice) -> Mux3/1, Sum1/1
  Constant/1 -> Add/1
  Add/1 -> smooth pipe heat exchanger/7(fract. of ice), Mux4/3  "fraction of ice"
  1/h_ice1/1 -> Saturation/1
  undisturbed ground temperature/1(Tearth) -> Sum3/2
  Mux4/1 -> data/1
  THVsource/1 -> Demux6/1
  Mux1/1 -> THV_source/1
  Demux6/3 -> Mux1/3, heat exchanger solar/3(mdot)  "mdot"
  Demux6/4 -> Mux1/4, heat exchanger solar/4(p)  "p"
  Demux6/5 -> Mux1/5, heat exchanger solar/5(fluid)  "fluid"
  Demux6/7 -> Mux1/7  "d clq other"
  Demux6/1 -> Mux1/1  "ID"
  Demux6/6 -> Mux1/6, heat exchanger solar/6(mix)  "mix"
  Demux6/2 -> heat exchanger solar/2(Tin)  "T"
  heat exchanger solar/2(Thx_coll) -> Mux1/2
  1/m/1 -> Integrator/1
  Sum1/1 -> 1/m/1
  Sum2/1 -> UAtank/1
  UAtank/1 -> Sum1/2, Sum4/1, Mux3/2  "Qdot_earth2ice"
  Integrator/1 -> 1/h_ice1/1, h 2 T/1  "h"
  Sum3/1 -> UAearth/1
  UAearth/1 -> Sum4/2
  Sum4/1 -> 1/m/cp/1
  1/m/cp/1 -> Integrator1/1
  Integrator1/1 -> Sum2/2, Sum3/1
  h 2 T/1 -> Mux4/1, Tice/1, Sum2/1, smooth pipe heat exchanger/1(Tice), heat exchanger solar/1(Tice)
  THVload/1 -> Demux1/1
  Mux2/1 -> THV_load/1
  Demux1/3 -> Mux2/3, smooth pipe heat exchanger/3(mdot)  "mdot"
  Demux1/4 -> Mux2/4, smooth pipe heat exchanger/4(p)  "p"
  Demux1/5 -> Mux2/5, smooth pipe heat exchanger/5(fluid)  "fluid"
  Demux1/7 -> Mux2/7  "d clq other"
  Demux1/1 -> Mux2/1  "ID"
  Demux1/6 -> smooth pipe heat exchanger/6(mix), Mux2/6  "mix"
  Demux1/2 -> smooth pipe heat exchanger/2(Tin)  "T"
  Mux3/1 -> Mux4/2
  Saturation/1 -> Add/2
  heat exchanger solar/1(Qdot2ice) -> Sum1/3, Mux3/3

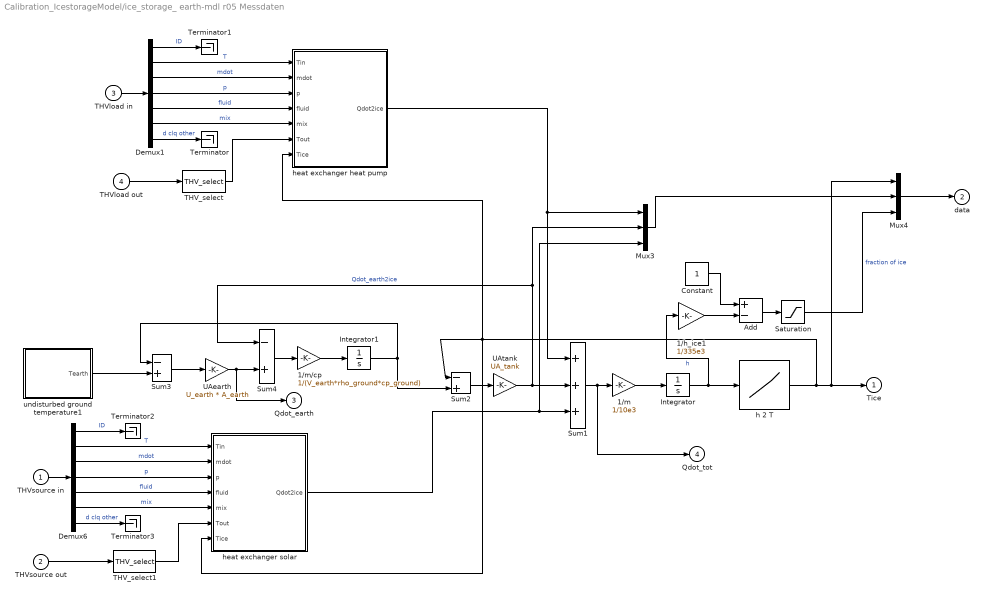
== system Calibration_IcestorageModel/ice_storage_ earth-mdl r05 Messdaten ==
  THVsource in : Inport
  THVsource out : Inport  Port=2
  THVload in : Inport  Port=3
  THVload out : Inport  Port=4
  1/h_ice1 : Gain  Gain=1/335e3  SaturateOnIntegerOverflow=on  OutDataTypeStr=Inherit: Same as input  ParamDataTypeStr=Inherit: Same as input
  1/m : Gain  Gain=1/10e3  SaturateOnIntegerOverflow=on  OutDataTypeStr=Inherit: Same as input  ParamDataTypeStr=Inherit: Same as input
  1/m/cp : Gain  Gain=1/(V_earth*rho_ground*cp_ground)  SaturateOnIntegerOverflow=on  OutDataTypeStr=Inherit: Same as input  ParamDataTypeStr=Inherit: Same as input
  Add : Sum  Inputs=+-
  Constant : Constant
  Demux1 : Demux  Outputs=[1 1 1 1 1 1 14]
  Demux6 : Demux  Outputs=[1 1 1 1 1 1 14]
  Integrator : Integrator  InitialCondition=h_ini
  Integrator1 : Integrator  InitialCondition=5
  Mux3 : Mux  Inputs=3
  Mux4 : Mux  Inputs=3
  Saturation : Saturate  UpperLimit=1  LowerLimit=0  LinearizeAsGain=off
  Sum1 : Sum  Inputs=+++  SaturateOnIntegerOverflow=on  InputSameDT=on  OutDataTypeStr=Inherit: Same as first input
  Sum2 : Sum  Inputs=-+  SaturateOnIntegerOverflow=on  InputSameDT=on  OutDataTypeStr=Inherit: Same as first input
  Sum3 : Sum  Inputs=-+  SaturateOnIntegerOverflow=on  InputSameDT=on  OutDataTypeStr=Inherit: Same as first input
  Sum4 : Sum  Inputs=-+  SaturateOnIntegerOverflow=on  InputSameDT=on  OutDataTypeStr=Inherit: Same as first input
  THV_select : carnot/Outputs/THV_select  f=off  t=on  m=off  p=off  id=off  mix=off  d=off  dpcon=off  dplin=off  dpqua=off
      settings: SourceProductName=Carnot
  THV_select1 : carnot/Outputs/THV_select  f=off  t=on  m=off  p=off  id=off  mix=off  d=off  dpcon=off  dplin=off  dpqua=off
      settings: SourceProductName=Carnot
  Terminator{,1..3} (4 alike) : Terminator
  UAearth : Gain  Gain=U_earth * A_earth  SaturateOnIntegerOverflow=on  OutDataTypeStr=Inherit: Same as input  ParamDataTypeStr=Inherit: Same as input
  UAtank : Gain  Gain=UA_tank  SaturateOnIntegerOverflow=on  OutDataTypeStr=Inherit: Same as input  ParamDataTypeStr=Inherit: Same as input
  h 2 T : Lookup  InputValues=[-2060*10 -2060*3 335e3 335e3+4182*10]  Table=[-10 -3 0 10]
  heat exchanger heat pump : Subsystem
  heat exchanger solar : Subsystem
  undisturbed ground temperature1 : Subsystem
  Tice : Outport  InitialOutput=0
  data : Outport  Port=2  InitialOutput=0
  Qdot_earth : Outport  Port=3  InitialOutput=0
  Qdot_tot : Outport  Port=4  InitialOutput=0
  wires:
  THV_select1/1 -> heat exchanger solar/6(Tout)
  THVsource out/1 -> THV_select1/1
  Demux6/7 -> Terminator3/1  "d clq other"
  Demux6/1 -> Terminator2/1  "ID"
  THVload out/1 -> THV_select/1
  THV_select/1 -> heat exchanger heat pump/6(Tout)
  Demux1/1 -> Terminator1/1  "ID"
  Demux1/7 -> Terminator/1  "d clq other"
  Mux3/1 -> Mux4/2
  heat exchanger heat pump/1(Qdot2ice) -> Mux3/1, Sum1/1
  Demux1/2 -> heat exchanger heat pump/1(Tin)  "T"
  Demux1/6 -> heat exchanger heat pump/5(mix)  "mix"
  Demux1/5 -> heat exchanger heat pump/4(fluid)  "fluid"
  Demux1/4 -> heat exchanger heat pump/3(p)  "p"
  Demux1/3 -> heat exchanger heat pump/2(mdot)  "mdot"
  THVload in/1 -> Demux1/1
  heat exchanger solar/1(Qdot2ice) -> Sum1/3, Mux3/3
  h 2 T/1 -> Mux4/1, Tice/1, Sum2/1, heat exchanger heat pump/7(Tice), heat exchanger solar/7(Tice)
  Integrator1/1 -> Sum3/1, Sum2/2
  1/m/cp/1 -> Integrator1/1
  Sum4/1 -> 1/m/cp/1
  UAearth/1 -> Sum4/2, Qdot_earth/1
  Sum3/1 -> UAearth/1
  Integrator/1 -> h 2 T/1, 1/h_ice1/1  "h"
  UAtank/1 -> Mux3/2, Sum4/1, Sum1/2  "Qdot_earth2ice"
  Sum2/1 -> UAtank/1
  Sum1/1 -> 1/m/1, Qdot_tot/1
  1/m/1 -> Integrator/1
  Demux6/2 -> heat exchanger solar/1(Tin)  "T"
  Demux6/6 -> heat exchanger solar/5(mix)  "mix"
  Demux6/5 -> heat exchanger solar/4(fluid)  "fluid"
  Demux6/4 -> heat exchanger solar/3(p)  "p"
  Demux6/3 -> heat exchanger solar/2(mdot)  "mdot"
  THVsource in/1 -> Demux6/1
  Mux4/1 -> data/1
  1/h_ice1/1 -> Add/2
  Add/1 -> Saturation/1
  Constant/1 -> Add/1
  Saturation/1 -> Mux4/3  "fraction of ice"
  undisturbed ground temperature1/1(Tearth) -> Sum3/2

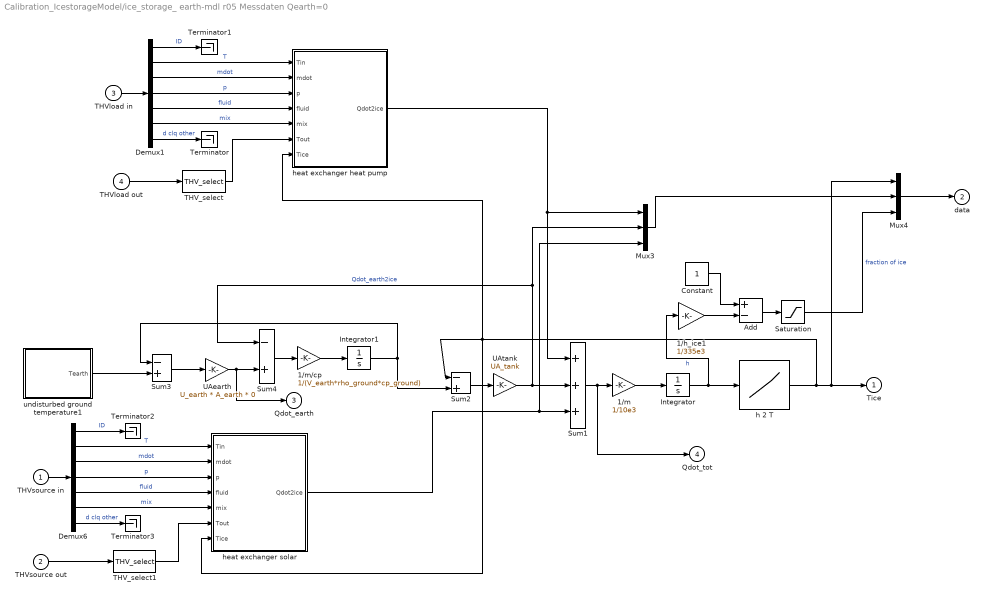
== system Calibration_IcestorageModel/ice_storage_ earth-mdl r05 Messdaten Qearth=0 ==
  THVsource in : Inport
  THVsource out : Inport  Port=2
  THVload in : Inport  Port=3
  THVload out : Inport  Port=4
  1/h_ice1 : Gain  Gain=1/335e3  SaturateOnIntegerOverflow=on  OutDataTypeStr=Inherit: Same as input  ParamDataTypeStr=Inherit: Same as input
  1/m : Gain  Gain=1/10e3  SaturateOnIntegerOverflow=on  OutDataTypeStr=Inherit: Same as input  ParamDataTypeStr=Inherit: Same as input
  1/m/cp : Gain  Gain=1/(V_earth*rho_ground*cp_ground)  SaturateOnIntegerOverflow=on  OutDataTypeStr=Inherit: Same as input  ParamDataTypeStr=Inherit: Same as input
  Add : Sum  Inputs=+-
  Constant : Constant
  Demux1 : Demux  Outputs=[1 1 1 1 1 1 14]
  Demux6 : Demux  Outputs=[1 1 1 1 1 1 14]
  Integrator : Integrator  InitialCondition=h_ini
  Integrator1 : Integrator  InitialCondition=5
  Mux3 : Mux  Inputs=3
  Mux4 : Mux  Inputs=3
  Saturation : Saturate  UpperLimit=1  LowerLimit=0  LinearizeAsGain=off
  Sum1 : Sum  Inputs=+++  SaturateOnIntegerOverflow=on  InputSameDT=on  OutDataTypeStr=Inherit: Same as first input
  Sum2 : Sum  Inputs=-+  SaturateOnIntegerOverflow=on  InputSameDT=on  OutDataTypeStr=Inherit: Same as first input
  Sum3 : Sum  Inputs=-+  SaturateOnIntegerOverflow=on  InputSameDT=on  OutDataTypeStr=Inherit: Same as first input
  Sum4 : Sum  Inputs=-+  SaturateOnIntegerOverflow=on  InputSameDT=on  OutDataTypeStr=Inherit: Same as first input
  THV_select : carnot/Outputs/THV_select  f=off  t=on  m=off  p=off  id=off  mix=off  d=off  dpcon=off  dplin=off  dpqua=off
      settings: SourceProductName=Carnot
  THV_select1 : carnot/Outputs/THV_select  f=off  t=on  m=off  p=off  id=off  mix=off  d=off  dpcon=off  dplin=off  dpqua=off
      settings: SourceProductName=Carnot
  Terminator{,1..3} (4 alike) : Terminator
  UAearth : Gain  Gain=U_earth * A_earth * 0  SaturateOnIntegerOverflow=on  OutDataTypeStr=Inherit: Same as input  ParamDataTypeStr=Inherit: Same as input
  UAtank : Gain  Gain=UA_tank  SaturateOnIntegerOverflow=on  OutDataTypeStr=Inherit: Same as input  ParamDataTypeStr=Inherit: Same as input
  h 2 T : Lookup  InputValues=[-2060*10 -2060*3 335e3 335e3+4182*10]  Table=[-10 -3 0 10]
  heat exchanger heat pump : Subsystem
  heat exchanger solar : Subsystem
  undisturbed ground temperature1 : Subsystem
  Tice : Outport  InitialOutput=0
  data : Outport  Port=2  InitialOutput=0
  Qdot_earth : Outport  Port=3  InitialOutput=0
  Qdot_tot : Outport  Port=4  InitialOutput=0
  wires:
  undisturbed ground temperature1/1(Tearth) -> Sum3/2
  Saturation/1 -> Mux4/3  "fraction of ice"
  Constant/1 -> Add/1
  Add/1 -> Saturation/1
  1/h_ice1/1 -> Add/2
  Mux4/1 -> data/1
  THVsource in/1 -> Demux6/1
  Demux6/3 -> heat exchanger solar/2(mdot)  "mdot"
  Demux6/4 -> heat exchanger solar/3(p)  "p"
  Demux6/5 -> heat exchanger solar/4(fluid)  "fluid"
  Demux6/6 -> heat exchanger solar/5(mix)  "mix"
  Demux6/2 -> heat exchanger solar/1(Tin)  "T"
  1/m/1 -> Integrator/1
  Sum1/1 -> Qdot_tot/1, 1/m/1
  Sum2/1 -> UAtank/1
  UAtank/1 -> Sum1/2, Sum4/1, Mux3/2  "Qdot_earth2ice"
  Integrator/1 -> 1/h_ice1/1, h 2 T/1  "h"
  Sum3/1 -> UAearth/1
  UAearth/1 -> Qdot_earth/1, Sum4/2
  Sum4/1 -> 1/m/cp/1
  1/m/cp/1 -> Integrator1/1
  Integrator1/1 -> Sum2/2, Sum3/1
  h 2 T/1 -> heat exchanger solar/7(Tice), heat exchanger heat pump/7(Tice), Sum2/1, Tice/1, Mux4/1
  heat exchanger solar/1(Qdot2ice) -> Sum1/3, Mux3/3
  THVload in/1 -> Demux1/1
  Demux1/3 -> heat exchanger heat pump/2(mdot)  "mdot"
  Demux1/4 -> heat exchanger heat pump/3(p)  "p"
  Demux1/5 -> heat exchanger heat pump/4(fluid)  "fluid"
  Demux1/6 -> heat exchanger heat pump/5(mix)  "mix"
  Demux1/2 -> heat exchanger heat pump/1(Tin)  "T"
  heat exchanger heat pump/1(Qdot2ice) -> Sum1/1, Mux3/1
  Mux3/1 -> Mux4/2
  Demux1/7 -> Terminator/1  "d clq other"
  Demux1/1 -> Terminator1/1  "ID"
  THV_select/1 -> heat exchanger heat pump/6(Tout)
  THVload out/1 -> THV_select/1
  Demux6/1 -> Terminator2/1  "ID"
  Demux6/7 -> Terminator3/1  "d clq other"
  THVsource out/1 -> THV_select1/1
  THV_select1/1 -> heat exchanger solar/6(Tout)

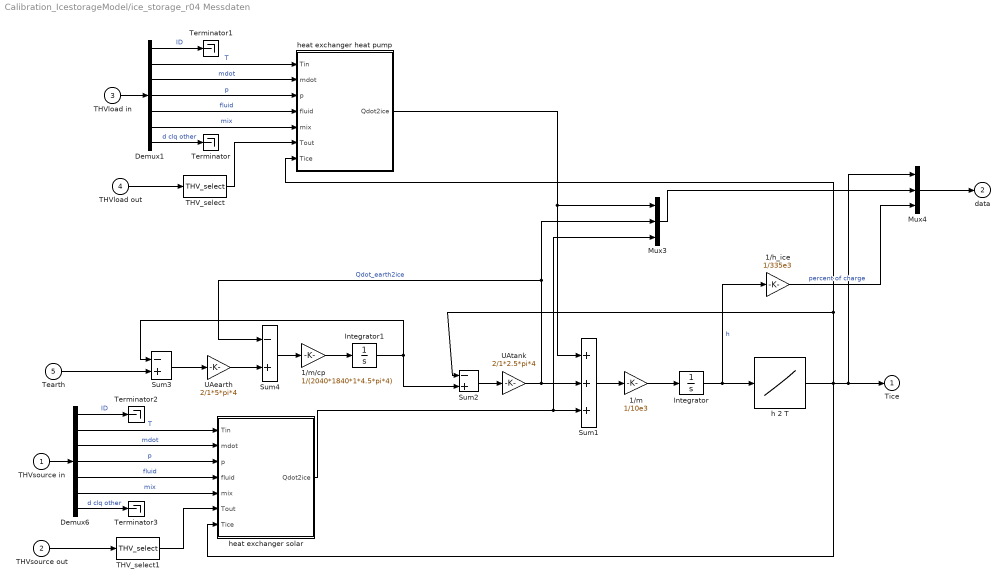
== system Calibration_IcestorageModel/ice_storage_r04 Messdaten ==
  THVsource in : Inport
  THVsource out : Inport  Port=2
  THVload in : Inport  Port=3
  THVload out : Inport  Port=4
  Tearth : Inport  Port=5
  1/h_ice : Gain  Gain=1/335e3  SaturateOnIntegerOverflow=on  OutDataTypeStr=Inherit: Same as input  ParamDataTypeStr=Inherit: Same as input
  1/m : Gain  Gain=1/10e3  SaturateOnIntegerOverflow=on  OutDataTypeStr=Inherit: Same as input  ParamDataTypeStr=Inherit: Same as input
  1/m/cp : Gain  Gain=1/(2040*1840*1*4.5*pi*4)  SaturateOnIntegerOverflow=on  OutDataTypeStr=Inherit: Same as input  ParamDataTypeStr=Inherit: Same as input
  Demux1 : Demux  Outputs=[1 1 1 1 1 1 14]
  Demux6 : Demux  Outputs=[1 1 1 1 1 1 14]
  Integrator : Integrator  InitialCondition=h_ini
  Integrator1 : Integrator  InitialCondition=5
  Mux3 : Mux  Inputs=3
  Mux4 : Mux  Inputs=3
  Sum1 : Sum  Inputs=+++  SaturateOnIntegerOverflow=on  InputSameDT=on  OutDataTypeStr=Inherit: Same as first input
  Sum2 : Sum  Inputs=-+  SaturateOnIntegerOverflow=on  InputSameDT=on  OutDataTypeStr=Inherit: Same as first input
  Sum3 : Sum  Inputs=-+  SaturateOnIntegerOverflow=on  InputSameDT=on  OutDataTypeStr=Inherit: Same as first input
  Sum4 : Sum  Inputs=-+  SaturateOnIntegerOverflow=on  InputSameDT=on  OutDataTypeStr=Inherit: Same as first input
  THV_select : carnot/Outputs/THV_select  f=off  t=on  m=off  p=off  id=off  mix=off  d=off  dpcon=off  dplin=off  dpqua=off
      settings: SourceProductName=Carnot
  THV_select1 : carnot/Outputs/THV_select  f=off  t=on  m=off  p=off  id=off  mix=off  d=off  dpcon=off  dplin=off  dpqua=off
      settings: SourceProductName=Carnot
  Terminator{,1..3} (4 alike) : Terminator
  UAearth : Gain  Gain=2/1*5*pi*4  SaturateOnIntegerOverflow=on  OutDataTypeStr=Inherit: Same as input  ParamDataTypeStr=Inherit: Same as input
  UAtank : Gain  Gain=2/1*2.5*pi*4  SaturateOnIntegerOverflow=on  OutDataTypeStr=Inherit: Same as input  ParamDataTypeStr=Inherit: Same as input
  h 2 T : Lookup  InputValues=[-2060*10 -2060*3 335e3 335e3+4182*10]  Table=[-10 -3 0 10]
  heat exchanger heat pump : Subsystem
  heat exchanger solar : Subsystem
  Tice : Outport  InitialOutput=0
  data : Outport  Port=2  InitialOutput=0
  wires:
  Mux3/1 -> Mux4/2
  heat exchanger heat pump/1(Qdot2ice) -> Mux3/1, Sum1/1
  heat exchanger solar/1(Qdot2ice) -> Mux3/3, Sum1/3
  Tearth/1 -> Sum3/2
  h 2 T/1 -> Sum2/1, heat exchanger heat pump/7(Tice), Tice/1, Mux4/1, heat exchanger solar/7(Tice)
  Integrator1/1 -> Sum3/1, Sum2/2
  1/m/cp/1 -> Integrator1/1
  Sum4/1 -> 1/m/cp/1
  UAearth/1 -> Sum4/2
  Sum3/1 -> UAearth/1
  Integrator/1 -> h 2 T/1, 1/h_ice/1  "h"
  UAtank/1 -> Mux3/2, Sum4/1, Sum1/2  "Qdot_earth2ice"
  Sum2/1 -> UAtank/1
  Sum1/1 -> 1/m/1
  1/m/1 -> Integrator/1
  Mux4/1 -> data/1
  1/h_ice/1 -> Mux4/3  "percent of charge"
  THVload out/1 -> THV_select/1
  THV_select/1 -> heat exchanger heat pump/6(Tout)
  Demux1/1 -> Terminator1/1  "ID"
  Demux1/7 -> Terminator/1  "d clq other"
  Demux1/2 -> heat exchanger heat pump/1(Tin)  "T"
  Demux1/6 -> heat exchanger heat pump/5(mix)  "mix"
  Demux1/5 -> heat exchanger heat pump/4(fluid)  "fluid"
  Demux1/4 -> heat exchanger heat pump/3(p)  "p"
  Demux1/3 -> heat exchanger heat pump/2(mdot)  "mdot"
  THVload in/1 -> Demux1/1
  THV_select1/1 -> heat exchanger solar/6(Tout)
  THVsource out/1 -> THV_select1/1
  Demux6/7 -> Terminator3/1  "d clq other"
  Demux6/1 -> Terminator2/1  "ID"
  Demux6/2 -> heat exchanger solar/1(Tin)  "T"
  Demux6/6 -> heat exchanger solar/5(mix)  "mix"
  Demux6/5 -> heat exchanger solar/4(fluid)  "fluid"
  Demux6/4 -> heat exchanger solar/3(p)  "p"
  Demux6/3 -> heat exchanger solar/2(mdot)  "mdot"
  THVsource in/1 -> Demux6/1

== system Calibration_IcestorageModel/Daten Ldf einlesen messdaten1_2011dez_2012aug/Heiz ==
  data : Inport
  Selector : Selector  InputPortWidth=36  IndexOptions=Index vector (dialog)  Indices=[v]  OutputSizes=1
  out : Outport  InitialOutput=0
  wires:
  data/1 -> Selector/1
  Selector/1 -> out/1
